simulink model "CicPLL"  (Simulink 6.3)
settings: Solver=FixedStepDiscrete  SolverMode=SingleTasking  StartTime=0.0  StopTime=3000*8*20e-9  RelTol=1e-3
InitFcn:
  | %% DSPBuilder Start
  | alt_dspbuilder_update_model(bdroot)
  | %% DSPBuilder End
StopFcn:
  | fftplot(input)
  | fftplot(output)
libraries: allblocks_alteradspbuilder2 x23
settings Model: Creator=mjervis  LastModifiedBy=LKONG
settings DataIOCC: SignalLoggingName=sigsOut
settings OptimizationCC: BooleanDataType=off  InlineInvariantSignals=on
settings DebuggingCC: SolverPrmCheckMsg=none
settings HardwareCC: TargetUnknown=on

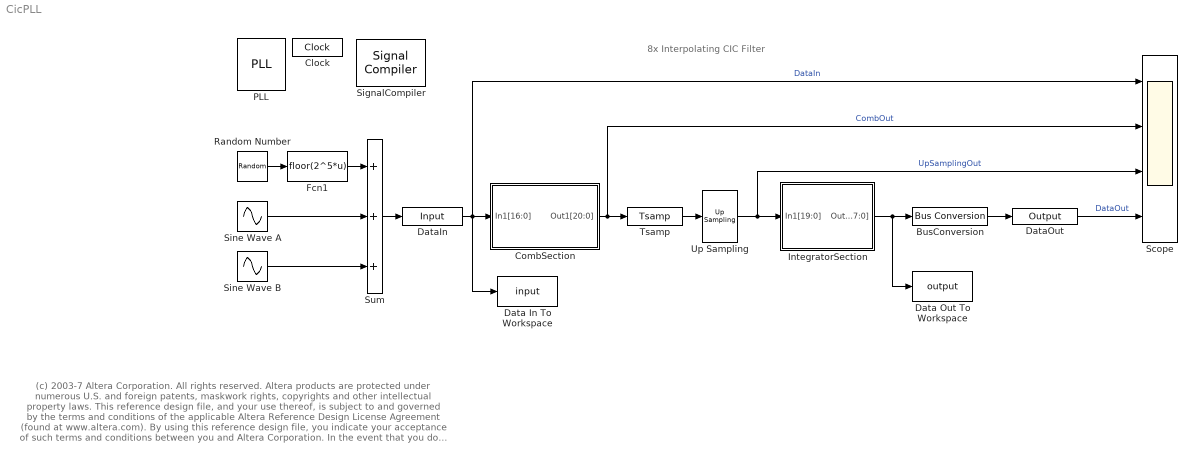
== system CicPLL ==
  note: 8x Interpolating CIC Filter
  note: (c) 2003-7 Altera Corporation. All rights reserved.  Altera products are protected under numerous U.S. and foreign patents, maskwork rights, copyrights and other intellectual property laws.
      | This reference design file, and your use thereof, is subject to and governed by the terms and conditions of the applicable Altera Reference Design License Agreement (found at www.altera.com).
      | By using this reference design file, you indicate your acceptance of such terms and conditions between you and Altera Corporation.
      | In the event that you do not agree with such terms and conditions, you may not use the reference design file and please promptly destroy any copies you have made.
      | This reference design file being provided on an "as-is" basis and as an accommodation and therefore all warranties, representations or guarantees of any kind (whether express, implied or statutory)
      | including, without limitation, warranties of merchantability, non-infringement, or fitness for a particular purpose, are specifically disclaimed.
      | By making this reference design file available, Altera expressly does not recommend, suggest or require that this reference design file be used in combination with any other product not provided by Altera
  BusConversion : allblocks_alteradspbuilder2/Bus Conversion  BusType=Signed Integer  ibwl=28  ibwr=0  bwl=16  bwr=0  bitToConnectToOutputLSB=12  round=off  saturate=off
  Clock : allblocks_alteradspbuilder2/Clock  ClockPeriod=160  ClockPeriodUnit=ns  SampleTime=160e-9  SimulationStartCycle=5  PhaseOffset=0  Reset=aclr  ResetType=Active Low  Export=off
  CombSection : Subsystem  AncestorBlock=ALTELINK/AltLab/HDL SubSystem
      mask Type: SubSystem AlteraBlockSet
  Data In To Workspace : ToWorkspace  VariableName=input  SampleTime=160e-9  SaveFormat=Array
  Data Out To Workspace : ToWorkspace  VariableName=output  SampleTime=-1  SaveFormat=Array
  DataIn : allblocks_alteradspbuilder2/Input  iofile=d:\wsTrunk\workspace\Documentation\DesignExamples\Demos\Filters\CicFilter\CicPLL\tb_CicPLL\CicPLL_DataIn.salt  BusType=Signed Integer  bwl=16  bwr=0  SpecifyClock=on  clock=PLL_clk1  PORTTYPE=Input
  DataOut : allblocks_alteradspbuilder2/Output  iofile=d:\wsTrunk\workspace\Documentation\DesignExamples\Demos\Filters\CicFilter\CicPLL\tb_CicPLL\CicPLL_DataOut.capture  BusType=Signed Integer  bwl=16  bwr=0  PORTTYPE=Output
  Fcn1 : Fcn  Expr=floor(2^5*u)
  IntegratorSection : Subsystem  AncestorBlock=ALTELINK/AltLab/HDL SubSystem
      mask Type: SubSystem AlteraBlockSet
  PLL : allblocks_alteradspbuilder2/PLL  clock_mult=[1, 1, 3, 4, 1, 1, 1, 1, 1]  clock_divide=[8, 1, 3, 1, 1, 1, 1, 1, 1]  clock_export=[0, 0, 0, 0, 0, 0, 0, 0, 0]  num_clocks=2  input_clock=Clock1  use_base_clock=on
  Random Number : RandomNumber  Variance=8  SampleTime=160e-9
  Scope : Scope  NumInputPorts=4
      settings: TimeRange=0.00012  YMin=-3000~-6000~-6000~-2000  YMax=3000~6000~6000~2000
  SignalCompiler : allblocks_alteradspbuilder2/Signal Compiler  DeviceFamily=Stratix III  DeviceName=AUTO  EnableSignalTap=off  SignalTapDepth=128  UseBoardBlock=off  StpUseDefaultClock=on  StpClock=clock
  Sine Wave A : Sin  SineType=Sample based  Amplitude=2^10-1  Samples=5  SampleTime=160e-9
  Sine Wave B : Sin  SineType=Sample based  Amplitude=2^10-1  Samples=500  SampleTime=160e-9
  Sum : Sum  Inputs=+++  SaturateOnIntegerOverflow=on  InputSameDT=on
  Tsamp : allblocks_alteradspbuilder2/Tsamp  SpecifyClock=on  clock=PLL_clk0
  Up Sampling : allblocks_alteradspbuilder2/Up Sampling  rate=8
  wires:
  Up Sampling/1 -> IntegratorSection/1(In1[19:0]), Scope/3  "UpSamplingOut"
  IntegratorSection/1(Out1[27:0]) -> Data Out To Workspace/1, BusConversion/1
  Random Number/1 -> Fcn1/1
  CombSection/1(Out1[20:0]) -> Tsamp/1, Scope/2  "CombOut"
  Tsamp/1 -> Up Sampling/1
  BusConversion/1 -> DataOut/1
  Fcn1/1 -> Sum/1
  Sine Wave A/1 -> Sum/2
  Sum/1 -> DataIn/1
  Sine Wave B/1 -> Sum/3
  DataOut/1 -> Scope/4  "DataOut"
  DataIn/1 -> CombSection/1(In1[16:0]), Scope/1, Data In To Workspace/1  "DataIn"

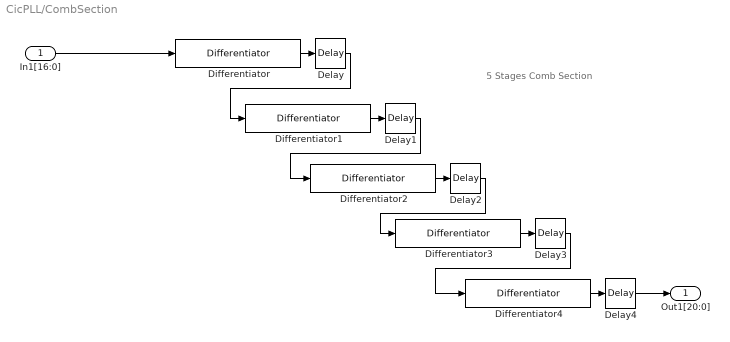
== system CicPLL/CombSection ==
  note: 5 Stages Comb Section
  In1[16:0] : Inport
  Delay{,1..4} (5 alike) : allblocks_alteradspbuilder2/Delay  pipeline=1  ClockPhase=1  use_ena=off  use_sclr=off  use_init=off  reset_value=1
  Differentiator : allblocks_alteradspbuilder2/Differentiator  bwl=17  depth=1  use_ena=off  use_sclr=off
  Differentiator1 : allblocks_alteradspbuilder2/Differentiator  bwl=18  depth=1  use_ena=off  use_sclr=off
  Differentiator2 : allblocks_alteradspbuilder2/Differentiator  bwl=19  depth=1  use_ena=off  use_sclr=off
  Differentiator3 : allblocks_alteradspbuilder2/Differentiator  bwl=20  depth=1  use_ena=off  use_sclr=off
  Differentiator4 : allblocks_alteradspbuilder2/Differentiator  bwl=21  depth=1  use_ena=off  use_sclr=off
  Out1[20:0] : Outport
  wires:
  In1[16:0]/1 -> Differentiator/1
  Delay4/1 -> Out1[20:0]/1
  Differentiator/1 -> Delay/1
  Differentiator1/1 -> Delay1/1
  Differentiator2/1 -> Delay2/1
  Differentiator3/1 -> Delay3/1
  Differentiator4/1 -> Delay4/1
  Delay/1 -> Differentiator1/1
  Delay1/1 -> Differentiator2/1
  Delay2/1 -> Differentiator3/1
  Delay3/1 -> Differentiator4/1

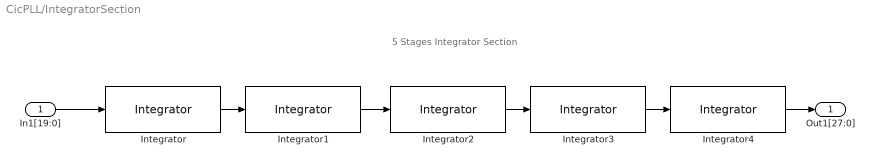
== system CicPLL/IntegratorSection ==
  note: 5 Stages Integrator Section
  In1[19:0] : Inport
  Integrator : allblocks_alteradspbuilder2/Integrator  bwl=20  depth=1  use_ena=off  use_sclr=off
  Integrator1 : allblocks_alteradspbuilder2/Integrator  bwl=22  depth=1  use_ena=off  use_sclr=off
  Integrator2 : allblocks_alteradspbuilder2/Integrator  bwl=24  depth=1  use_ena=off  use_sclr=off
  Integrator3 : allblocks_alteradspbuilder2/Integrator  bwl=26  depth=1  use_ena=off  use_sclr=off
  Integrator4 : allblocks_alteradspbuilder2/Integrator  bwl=28  depth=1  use_ena=off  use_sclr=off
  Out1[27:0] : Outport
  wires:
  In1[19:0]/1 -> Integrator/1
  Integrator/1 -> Integrator1/1
  Integrator1/1 -> Integrator2/1
  Integrator2/1 -> Integrator3/1
  Integrator3/1 -> Integrator4/1
  Integrator4/1 -> Out1[27:0]/1
